simulink model "SignalProcessing"  (R2026a)
settings: Solver=VariableStepAuto
undefined symbols (not defined in the file or in its folder): fs
libraries: dspfdesign x1
settings Model: Creator=UmarMuslimBinMohdFay  LastModifiedBy=UmarMuslimBinMohdFay

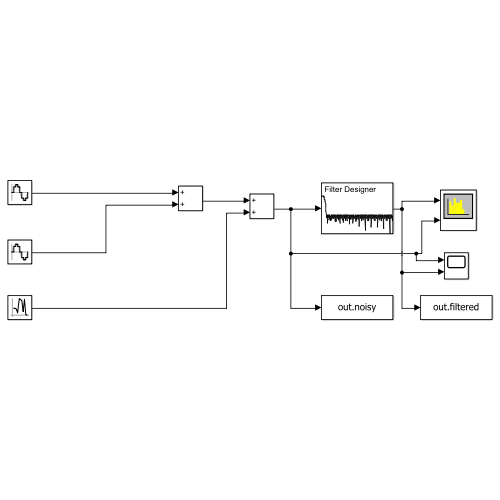
[thumbnail: Simulink's stored preview of the top-level diagram]
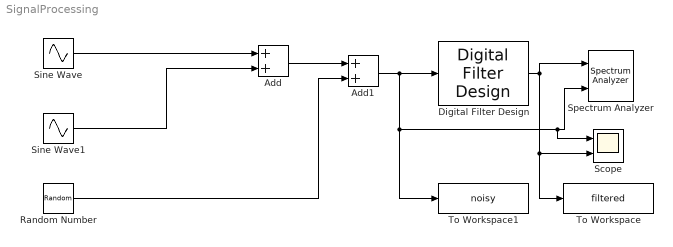
== system SignalProcessing ==
  Add : Sum
  Add1 : Sum
  Digital Filter Design : dspfdesign/Digital Filter Design  mwdsp_browser_bugfix_var=off
  Random Number : RandomNumber  Variance=0.4^2  SampleTime=1/fs
  Scope : Scope  NumInputPorts=2
      settings: ActiveDisplayYMinimum=-3.3137802715765932  ActiveDisplayYMaximum=3.1271103187311837
  Sine Wave : Sin  Frequency=2*pi*5  SampleTime=1/fs
  Sine Wave1 : Sin  Amplitude=0.5  Frequency=2*pi*40  SampleTime=1/fs
  Spectrum Analyzer : SpectrumAnalyzer  NumInputPorts=2  WindowPosition=[623.000000,1326.000000,800.000000,500.000000,]  Visible=on  ScopeFrameLocation=window  PlotAsTwoSidedSpectrum=off  WindowInvariantSamplesPerUpdate=on  Span=1000  StartFrequency=-500  StopFrequency=500  YLimits=[-50.5687 34.897]  SelectedToolstripTab=spectrumAnalyzerToolstrip.spectrumTab
  To Workspace : ToWorkspace  VariableName=filtered  SaveFormat=Timeseries  SampleTime=-1
  To Workspace1 : ToWorkspace  VariableName=noisy  SaveFormat=Timeseries  SampleTime=-1
  wires:
  Sine Wave/1 -> Add/1
  Sine Wave1/1 -> Add/2
  Add/1 -> Add1/1
  Random Number/1 -> Add1/2
  Add1/1 -> Scope/1, Spectrum Analyzer/2, To Workspace1/1, Digital Filter Design/1
  Digital Filter Design/1 -> Scope/2, To Workspace/1, Spectrum Analyzer/1
